simulink model "Sim1"  (R2020a)
settings: Solver=VariableStepAuto  StartTime=0.0  StopTime=0.05  RelTol=1e-5
values from neighbouring files (symbols this model uses):
  Kf = (R12+R8)/(R5+R8)    (= 1.32450331126)    [Main.m]
  Kg = 2*Km*Ubat    (= 48)    [Main.m]
  Tau1 = ((R8*R5)/(R8+R5))*C2    (= 7.43046357616e-05)    [Main.m]
  Tau2 = R21*C7    (= 4.84e-06)    [Main.m]
  tauc1 = Taum    (= 0.002)    [Main.m]
  tauc2 = 0.00268    [Main.m]
  Taum = Lm/Rm    (= 0.002)    [Main.m]
settings Model: Creator=belafki  LastModifiedBy=belafki

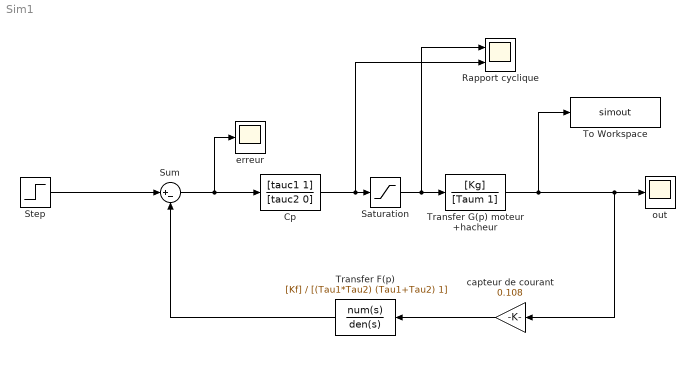
== system Sim1 ==
  Cp : TransferFcn  Numerator=[tauc1 1]  Denominator=[tauc2 0]
  Rapport cyclique : Scope  NumInputPorts=2
  Saturation : Saturate
  Step : Step  Time=0.01  After=1.65  SampleTime=0
  Sum : Sum  Inputs=|+-
  To Workspace : ToWorkspace  VariableName=simout  SaveFormat=Timeseries  SampleTime=-1
  Transfer F(p) : TransferFcn  Numerator=[Kf]  Denominator=[(Tau1*Tau2) (Tau1+Tau2) 1]
  Transfer G(p) moteur +hacheur : TransferFcn  Numerator=[Kg]  Denominator=[Taum 1]
  capteur de courant : Gain  Gain=0.108
  erreur : Scope
  out : Scope
  wires:
  Transfer G(p) moteur +hacheur/1 -> To Workspace/1, capteur de courant/1, out/1
  Transfer F(p)/1 -> Sum/2
  Step/1 -> Sum/1
  capteur de courant/1 -> Transfer F(p)/1
  Sum/1 -> erreur/1, Cp/1
  Cp/1 -> Rapport cyclique/2, Saturation/1
  Saturation/1 -> Rapport cyclique/1, Transfer G(p) moteur +hacheur/1
